simulink library "ECGAnalysisLib"  (R2020b)
settings: Solver=VariableStepAuto  StartTime=0.0  StopTime=10.0  RelTol=1e-3
undefined symbols (not defined in the file or in its folder): fs, max_hr, max_rr_dev
libraries: $bdroot x3
settings Model: Creator=Rafael  LastModifiedBy=Rafael

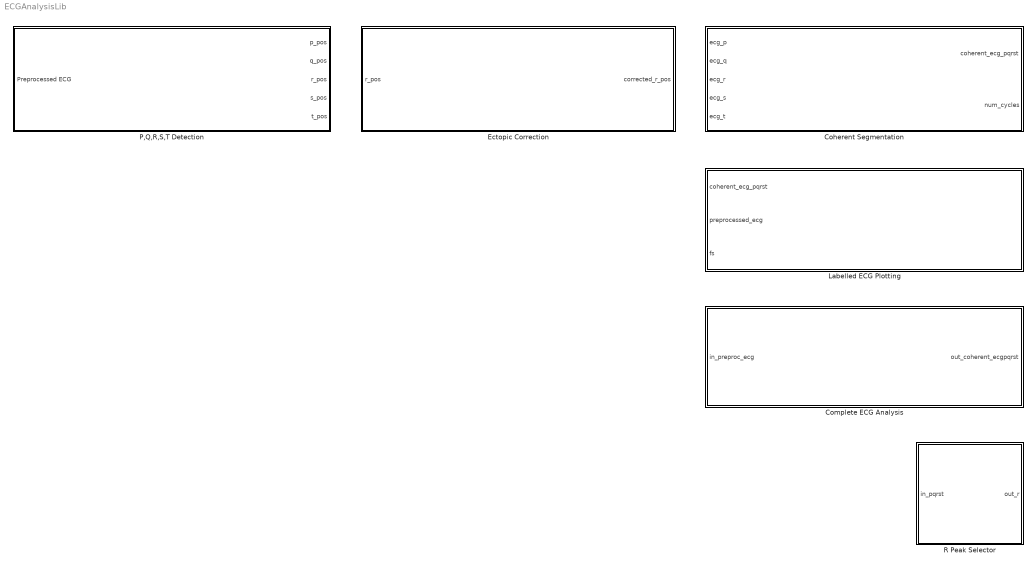
== system ECGAnalysisLib ==
  Coherent Segmentation : Subsystem
      mask Display: image('$imagefile'); % Use "Edit Image" on toolstrip to change.
  Complete ECG Analysis : Subsystem
      mask Display: image('$imagefile'); % Use "Edit Image" on toolstrip to change.
  Ectopic Correction : Subsystem
      mask Display: image('Tachogram.jpg'); % Use "Edit Image" on toolstrip to change.
  Labelled ECG Plotting : MATLAB Function  TreatAsAtomicUnit=on
  P,Q,R,S,T Detection : Subsystem  mask{ecg_algo=PQRST waves - Multi-level Teager Energy Operator}
      mask prompts: ecg_algo "Choose one:"
      mask init:
      | if ecg_algo == 1
      |     param_ecg_algo = 'Pan-Tompkins';
      | elseif ecg_algo == 2
      |     param_ecg_algo = 'Phase Space';
      | elseif ecg_algo == 3
      |     param_ecg_algo = 'Filter Bank';
      | elseif ecg_algo == 4
      |     param_ecg_algo = 'State Machine';
      | elseif ecg_algo == 5
      |     param_ecg_algo = 'Multi-level Teager Energy Operator';
      | end
      | 
      | assignin('base','param_ecg_algo', param_ecg_algo)
      mask TypeOptions ecg_algo: R wave  - Pan-Tompkins | R wave - Phase space | R wave - Filter bank | QRST waves - State machine | PQRST waves - Multi-level Teager Energy Operator
      mask DialogControl DescGroupVar Prompt: ECG PQRST Detection
      mask DialogControl DescTextVar Prompt: Select detected waveform(s) and corresponding detection aglorithm.
      mask DialogControl ParameterGroupVar Prompt: Desired wave(s) and Algorithm
      mask Display: image('$imagefile'); % Use "Edit Image" on toolstrip to change.
  R Peak Selector : Subsystem
      mask Display: image('$imagefile'); % Use "Edit Image" on toolstrip to change.

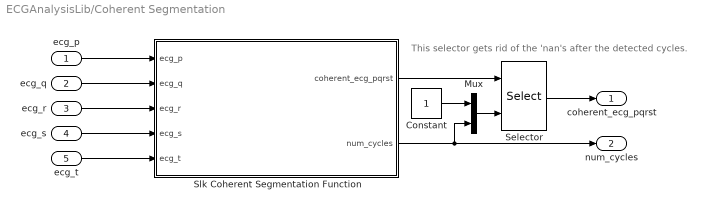
== system ECGAnalysisLib/Coherent Segmentation ==
  note: This selector gets rid of the 'nan's after the detected cycles.
  ecg_p : Inport
  ecg_q : Inport  Port=2
  ecg_r : Inport  Port=3
  ecg_s : Inport  Port=4
  ecg_t : Inport  Port=5
  Constant : Constant
  Mux : Mux  Inputs=2
  Selector : Selector  NumberOfDimensions=2  InputPortWidth=3  IndexOptions=Starting and ending indices (port),Index vector (dialog)  Indices=[1 3],[1 2 3 3 5]  OutputSizes=1,1
  Slk Coherent Segmentation Function : MATLAB Function  TreatAsAtomicUnit=on
  coherent_ecg_pqrst : Outport
  num_cycles : Outport  Port=2
  wires:
  ecg_q/1 -> Slk Coherent Segmentation Function/2(ecg_q)
  ecg_s/1 -> Slk Coherent Segmentation Function/4(ecg_s)
  ecg_p/1 -> Slk Coherent Segmentation Function/1(ecg_p)
  ecg_r/1 -> Slk Coherent Segmentation Function/3(ecg_r)
  ecg_t/1 -> Slk Coherent Segmentation Function/5(ecg_t)
  Constant/1 -> Mux/1
  Mux/1 -> Selector/2
  Slk Coherent Segmentation Function/1(coherent_ecg_pqrst) -> Selector/1
  Selector/1 -> coherent_ecg_pqrst/1
  Slk Coherent Segmentation Function/2(num_cycles) -> num_cycles/1, Mux/2

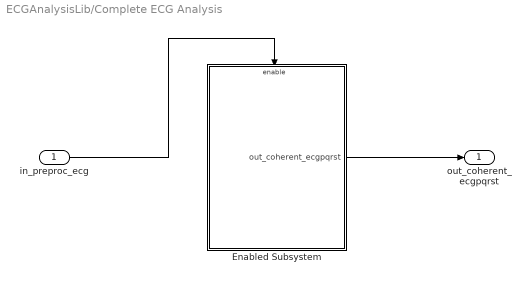
== system ECGAnalysisLib/Complete ECG Analysis ==
  in_preproc_ecg : Inport
  Enabled Subsystem : Subsystem  TreatAsAtomicUnit=on
  out_coherent_ecgpqrst : Outport
  wires:
  Enabled Subsystem/1(out_coherent_ecgpqrst) -> out_coherent_ecgpqrst/1
  in_preproc_ecg/1 -> Enabled Subsystem/Enable

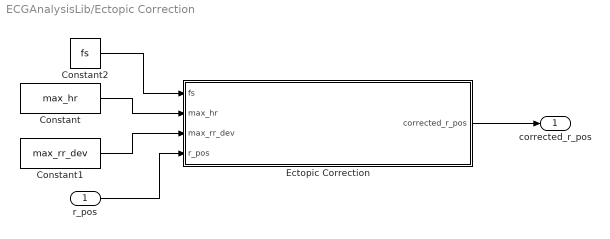
== system ECGAnalysisLib/Ectopic Correction ==
  r_pos : Inport
  Constant : Constant  Value=max_hr
  Constant1 : Constant  Value=max_rr_dev
  Constant2 : Constant  Value=fs
  Ectopic Correction : MATLAB Function  TreatAsAtomicUnit=on
  corrected_r_pos : Outport
  wires:
  r_pos/1 -> Ectopic Correction/4(r_pos)
  Ectopic Correction/1(corrected_r_pos) -> corrected_r_pos/1
  Constant2/1 -> Ectopic Correction/1(fs)
  Constant/1 -> Ectopic Correction/2(max_hr)
  Constant1/1 -> Ectopic Correction/3(max_rr_dev)

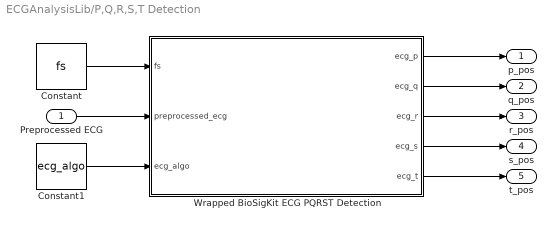
== system ECGAnalysisLib/P,Q,R,S,T Detection ==
  Preprocessed ECG : Inport
  Constant : Constant  Value=fs
  Constant1 : Constant  Value=ecg_algo
  Wrapped BioSigKit ECG PQRST Detection : MATLAB Function  TreatAsAtomicUnit=on
  p_pos : Outport
      settings: VarSizeSig=Yes
  q_pos : Outport  Port=2
      settings: VarSizeSig=Yes
  r_pos : Outport  Port=3
      settings: VarSizeSig=Yes
  s_pos : Outport  Port=4
      settings: VarSizeSig=Yes
  t_pos : Outport  Port=5
      settings: VarSizeSig=Yes
  wires:
  Preprocessed ECG/1 -> Wrapped BioSigKit ECG PQRST Detection/2(preprocessed_ecg)
  Constant/1 -> Wrapped BioSigKit ECG PQRST Detection/1(fs)
  Wrapped BioSigKit ECG PQRST Detection/1(ecg_p) -> p_pos/1
  Wrapped BioSigKit ECG PQRST Detection/2(ecg_q) -> q_pos/1
  Wrapped BioSigKit ECG PQRST Detection/3(ecg_r) -> r_pos/1
  Wrapped BioSigKit ECG PQRST Detection/4(ecg_s) -> s_pos/1
  Wrapped BioSigKit ECG PQRST Detection/5(ecg_t) -> t_pos/1
  Constant1/1 -> Wrapped BioSigKit ECG PQRST Detection/3(ecg_algo)

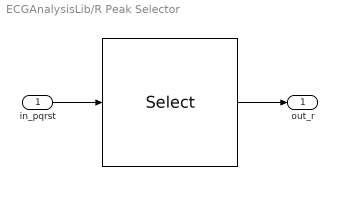
== system ECGAnalysisLib/R Peak Selector ==
  in_pqrst : Inport
  " " : Selector  NumberOfDimensions=2  InputPortWidth=3  IndexOptions=Select all,Index vector (dialog)  Indices=[1 3],3  OutputSizes=1,1
  out_r : Outport
  wires:
  in_pqrst/1 -> " "/1
  " "/1 -> out_r/1

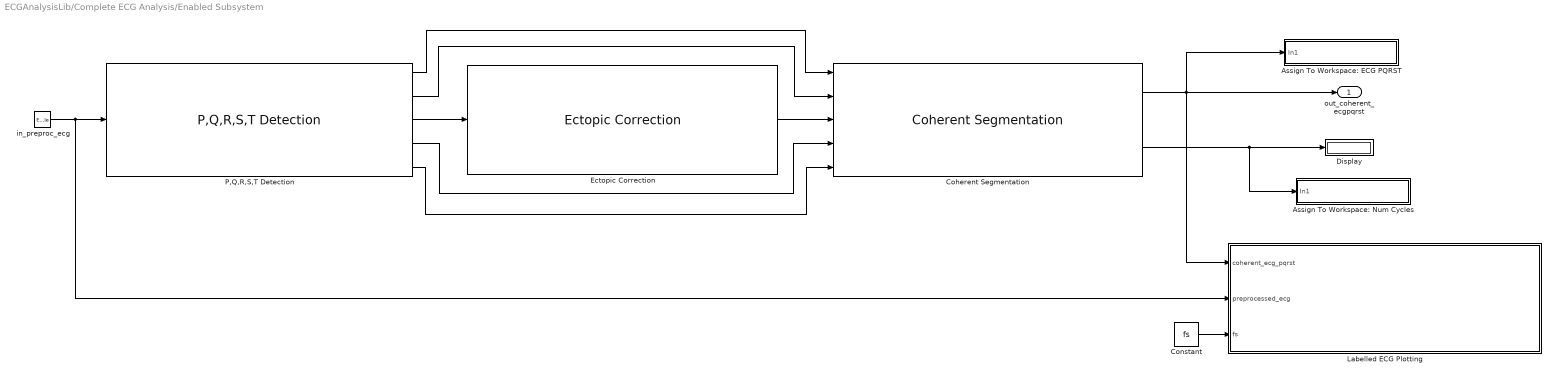
== system ECGAnalysisLib/Complete ECG Analysis/Enabled Subsystem ==
  in_preproc_ecg : EnablePort  ShowOutputPort=on
  Assign To Workspace: ECG PQRST : Subsystem
      mask Display: disp('Assign: out_ecg_pqrst')
  Assign To Workspace: Num Cycles : Subsystem
      mask Display: disp('Assign: out_ecg_num_cycles')
  Coherent Segmentation : $bdroot/Coherent Segmentation  SystemSampleTime=-1  VariantActivationTime=update diagram  Latency=0  AutoFrameSizeCalculation=off
  Constant : Constant  Value=fs
  Display : Display
  Ectopic Correction : $bdroot/Ectopic Correction  SystemSampleTime=-1  VariantActivationTime=update diagram  Latency=0  AutoFrameSizeCalculation=off
  Labelled ECG Plotting : MATLAB Function  TreatAsAtomicUnit=on
  P,Q,R,S,T Detection : $bdroot/P,Q,R,S,T Detection  ecg_algo=PQRST waves - Multi-level Teager Energy Operator
  out_coherent_ecgpqrst : Outport
  wires:
  P,Q,R,S,T Detection/3 -> Ectopic Correction/1
  Ectopic Correction/1 -> Coherent Segmentation/3
  P,Q,R,S,T Detection/1 -> Coherent Segmentation/1
  P,Q,R,S,T Detection/2 -> Coherent Segmentation/2
  P,Q,R,S,T Detection/4 -> Coherent Segmentation/4
  P,Q,R,S,T Detection/5 -> Coherent Segmentation/5
  in_preproc_ecg/1 -> Labelled ECG Plotting/2(preprocessed_ecg), P,Q,R,S,T Detection/1
  Constant/1 -> Labelled ECG Plotting/3(fs)
  Coherent Segmentation/1 -> Assign To Workspace: ECG PQRST/1(In1), Labelled ECG Plotting/1(coherent_ecg_pqrst), out_coherent_ecgpqrst/1
  Coherent Segmentation/2 -> Assign To Workspace: Num Cycles/1(In1), Display/1

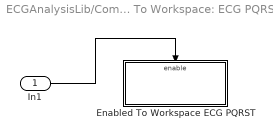
== system ECGAnalysisLib/Complete ECG Analysis/Enabled Subsystem/Assign To Workspace: ECG PQRST ==
  In1 : Inport
  Enabled To Workspace ECG PQRST : Subsystem  TreatAsAtomicUnit=on
  wires:
  In1/1 -> Enabled To Workspace ECG PQRST/Enable

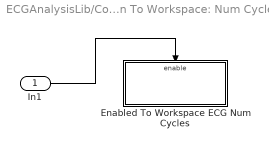
== system ECGAnalysisLib/Complete ECG Analysis/Enabled Subsystem/Assign To Workspace: Num Cycles ==
  In1 : Inport
  Enabled To Workspace ECG Num Cycles : Subsystem  TreatAsAtomicUnit=on
  wires:
  In1/1 -> Enabled To Workspace ECG Num Cycles/Enable

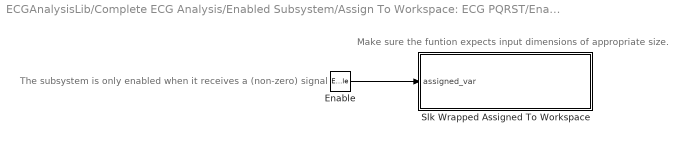
== system ECGAnalysisLib/Complete ECG Analysis/Enabled Subsystem/Assign To Workspace: ECG PQRST/Enabled To Workspace ECG PQRST ==
  note: Make sure the funtion expects input dimensions of appropriate size.
  note: The subsystem is only enabled when it receives a (non-zero) signal
  Enable : EnablePort  ShowOutputPort=on
  Slk Wrapped Assigned To Workspace : MATLAB Function  TreatAsAtomicUnit=on
  wires:
  Enable/1 -> Slk Wrapped Assigned To Workspace/1(assigned_var)

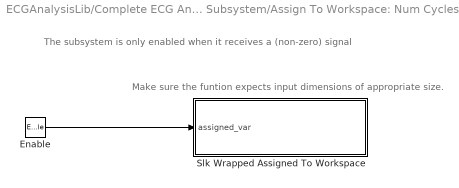
== system ECGAnalysisLib/Complete ECG Analysis/Enabled Subsystem/Assign To Workspace: Num Cycles/Enabled To Workspace ECG Num Cycles ==
  note: The subsystem is only enabled when it receives a (non-zero) signal
  note: Make sure the funtion expects input dimensions of appropriate size.
  Enable : EnablePort  ShowOutputPort=on
  Slk Wrapped Assigned To Workspace : MATLAB Function  TreatAsAtomicUnit=on
  wires:
  Enable/1 -> Slk Wrapped Assigned To Workspace/1(assigned_var)

== matlab function ECGAnalysisLib/Coherent Segmentation/Slk Coherent Segmentation Function ==
  data: ecg_p input size=[4*ceil(param_sim_time) 1]; coherent_ecg_pqrst output size=[4*ceil(param_sim_time) 5]; ecg_q input size=[4*ceil(param_sim_time) 1]; ecg_r input size=[4*ceil(param_sim_time) 1]; ecg_s input size=[4*ceil(param_sim_time) 1]; ecg_t input size=[4*ceil(param_sim_time) 1]; num_cycles output size=1
function [coherent_ecg_pqrst, num_cycles] = slk_coherent_segmentation(ecg_p, ecg_q, ecg_r, ecg_s, ecg_t)
% Function to associate the detected PQRST peaks to each other in a
% coherent way. The function will produce an output 'coherent_ecg_pqrst' of
% size [num_cycles x 5]. The 5 corresponds to the 5 fiducial points (PQRST
% peaks). num_cycles is the number of detected R peaks (heart cycles). The
% first column of coherent_ecg_prqst corresponds to the detected P waves,
% where the row corresponds to that cycle number. If a P wave couldnt be
% detected for that cycle, it is replaced with 'Nan'.


if ecg_r % Only go into the function if a valid ecg R peak sequence is passed to it.
    
    % Preinitialization.
    coherent_ecg_p = zeros(length(ecg_r),1);
    coherent_ecg_q = zeros(length(ecg_r),1);
    coherent_ecg_r = zeros(length(ecg_r),1);
    coherent_ecg_s = zeros(length(ecg_r),1);
    coherent_ecg_t = zeros(length(ecg_r),1);
        
    %% First Cycle.
    
    % P Wave.
    temp = ecg_p(find(ecg_p < ecg_r(1)));
    if isempty(temp)
        coherent_ecg_p(1) = nan;
        temp = [];
    else
        coherent_ecg_p(1) = temp;
    end
    
    % Q Wave.
    temp = ecg_p(find(ecg_q < ecg_r(1)));
    if isempty(temp)
        coherent_ecg_q(1) = nan;
        temp = [];
    else
        coherent_ecg_q(1) = temp;
    end
    
    % R Wave.
    coherent_ecg_r(1) = ecg_r(1);
    
    % S Wave.
    temp = ecg_s(find(ecg_s > ecg_r(1) & ecg_s < ecg_r(2)));
    if isempty(temp)
        coherent_ecg_s(1) = nan;
        temp = [];
    else
        coherent_ecg_s(1) = temp;
    end
    
    % T Wave.
    temp = ecg_t(find(ecg_t > ecg_r(1) & ecg_t < ecg_r(2)));
    if isempty(temp)
        coherent_ecg_t(1) = nan;
        temp = [];
    else
        coherent_ecg_t(1) = temp;
    end
    
    %% Cycle 2:End-1.
    for i = 2:length(ecg_r)-1
        
        % P Wave.
        temp = ecg_p(find(ecg_p > ecg_r(i-1) & ecg_p < ecg_r(i)));
        if isempty(temp) || length(temp) > 1
            coherent_ecg_p(i) = nan;
            temp = [];
        else
            coherent_ecg_p(i) = temp;
        end
        
        % Q Wave.
        temp = ecg_q(find(ecg_q > ecg_r(i-1) & ecg_q < ecg_r(i)));
        if isempty(temp) || length(temp) > 1
            coherent_ecg_q(i) = nan;
            temp = [];
        else
            coherent_ecg_q(i) = temp;
        end
        
        % R Wave.
        coherent_ecg_r(i) = ecg_r(i);
        
        % S Wave.
        temp = ecg_s(find(ecg_s > ecg_r(i) & ecg_s < ecg_r(i+1)));
        if isempty(temp) || length(temp) > 1
            coherent_ecg_s(i) = nan;
            temp = [];
        else
            coherent_ecg_s(i) = temp;
        end
        
        % T Wave.
        temp = ecg_t(find(ecg_t > ecg_r(i) & ecg_t < ecg_r(i+1)));
        if isempty(temp) || length(temp) > 1
            coherent_ecg_t(i) = nan;
            temp = [];
        else
            coherent_ecg_t(i) = temp;
        end
    end
    
    %% Last Cycle.
    
    % P Wave.
    temp = ecg_p(find(ecg_p > ecg_r(end-1) & ecg_p < ecg_r(end)));
    if isempty(temp) || length(temp) > 1
        coherent_ecg_p(length(ecg_r)) = nan;
        temp = [];
    else
        coherent_ecg_p(length(ecg_r)) = temp;
    end
    
    % Q Wave.
    temp = ecg_q(find(ecg_q > ecg_r(end-1) & ecg_q < ecg_r(end)));
    if isempty(temp) || length(temp) > 1
        coherent_ecg_q(length(ecg_r)) = nan;
        temp = [];
    else
        coherent_ecg_q(length(ecg_r)) = temp;
    end
    
    % R Wave.
    coherent_ecg_r(length(ecg_r)) = ecg_r(length(ecg_r));
    
    % S Wave.
    temp = ecg_s(find(ecg_s > ecg_r(1) & ecg_s < ecg_r(2)));
    if isempty(temp) || length(temp) > 1
        coherent_ecg_s(length(ecg_r)) = nan;
        temp = [];
    else
        coherent_ecg_s(length(ecg_r)) = temp;
    end
    
    % T Wave.
    temp = ecg_t(find(ecg_t > ecg_r(1) & ecg_t < ecg_r(2)));
    if isempty(temp) || length(temp) > 1
        coherent_ecg_t(length(ecg_r)) = nan;
        temp = [];
    else
        coherent_ecg_t(length(ecg_r)) = temp;
    end
    
    coherent_ecg_pqrst = [coherent_ecg_p coherent_ecg_q coherent_ecg_r coherent_ecg_s coherent_ecg_t];
    num_cycles = length(coherent_ecg_r);  
    
else
    
    coherent_ecg_pqrst = [];
    num_cycles = 0;
end
end

== matlab function ECGAnalysisLib/Labelled ECG Plotting ==
  data: coherent_ecg_pqrst input size=[4*ceil(param_sim_time) 5]; preprocessed_ecg input size=[param_tot_samples 1]; fs input size=[1]
function slk_wrapped_plotting_ecg_pqrst(coherent_ecg_pqrst, preprocessed_ecg, fs)
    
coder.extrinsic('plotting_ecg_pqrst');

if coherent_ecg_pqrst(:,3) % Only go into the function if a valid ecg R peak sequence is passed to it.
    plotting_ecg_pqrst(coherent_ecg_pqrst, preprocessed_ecg, fs)
end

end

== matlab function ECGAnalysisLib/Complete ECG Analysis/Enabled Subsystem/Labelled ECG Plotting ==
  data: coherent_ecg_pqrst input size=[4*ceil(param_sim_time) 5]; preprocessed_ecg input size=[param_tot_samples 1]; fs input size=[1]
function slk_wrapped_plotting_ecg_pqrst(coherent_ecg_pqrst, preprocessed_ecg, fs)
    
coder.extrinsic('plotting_ecg_pqrst');

if coherent_ecg_pqrst(:,3) % Only go into the function if a valid ecg R peak sequence is passed to it.
    plotting_ecg_pqrst(coherent_ecg_pqrst, preprocessed_ecg, fs)
end

end

== matlab function ECGAnalysisLib/Complete ECG Analysis/Enabled Subsystem/Assign To Workspace: ECG PQRST/Enabled To Workspace ECG PQRST/Slk Wrapped Assigned To Workspace ==
  data: assigned_var input size=[1]
function slk_wrapped_assign_to_workspace(assigned_var)
% Wrapped simulink function to assign an input 'assigned_var' to the base workspace.

coder.extrinsic('assign_num_cycles_to_workspace');

if assigned_var % Only go into the function if a valid variable is passed to it.
    assign_num_cycles_to_workspace(assigned_var)
end

end

== matlab function ECGAnalysisLib/P,Q,R,S,T Detection/Wrapped BioSigKit ECG PQRST Detection ==
  data: ecg_p output size=[4*ceil(param_sim_time) 1]; ecg_q output size=[4*ceil(param_sim_time) 1]; ecg_r output size=[4*ceil(param_sim_time) 1]; ecg_s output size=[4*ceil(param_sim_time) 1]; ecg_t output size=[4*ceil(param_sim_time) 1]; fs input; preprocessed_ecg input; ecg_algo input
function [ecg_p, ecg_q, ecg_r, ecg_s, ecg_t] = slk_wrapped_BioSigKit_ECG_Detection(fs, preprocessed_ecg, ecg_algo)

% This function is split in two parts out of necessity - (Simulink is kind of dumb).
% The first part counts how many detected P,Q,R,S, and T waves there are according to the BioSigKit method.
% With these numbers we can pre-initialize the size of the vectors holding the sample positions of these P,Q,R,S, and T waves which are then
% identified using a second identical use of the BioSigKit detection method.

coder.extrinsic('BioSigKit_ECG_Count_Detection');
coder.extrinsic('BioSigKit_ECG_Peak_Detection');

if preprocessed_ecg % The function is only run if a non-zero signal is passed to it.
    %% Part 1 - P,Q,R,S,T Count
    num_p = -1; % Pre-Initialization.
    num_q = -1;
    num_r = -1;
    num_s = -1;
    num_t = -1;
    
    [num_p, num_q, num_r, num_s, num_t] = BioSigKit_ECG_Count_Detection(fs,preprocessed_ecg, ecg_algo);
    
    %% Part 2 - P,Q,R,S,T Peak Identification
    ecg_p = zeros(num_p,1); % Pre-Initialization.
    ecg_q = zeros(num_q,1);
    ecg_r = zeros(num_r,1);
    ecg_s = zeros(num_s,1);
    ecg_t = zeros(num_t,1);
    
    % Performing the detection according to the desired detection algorithm.
    if ecg_algo == 1  || ecg_algo == 2 || ecg_algo == 3
        
        [~, ~, ecg_r(1:num_r), ~, ~] = BioSigKit_ECG_Peak_Detection(fs,preprocessed_ecg, ecg_algo);
        ecg_p = nan; ecg_q = nan; ecg_s = nan; ecg_t = nan;
        
    elseif ecg_algo == 4
        
        [~, ecg_q(1:num_q), ecg_r(1:num_r), ecg_s(1:num_s), ecg_t(1:num_t)] = BioSigKit_ECG_Peak_Detection(fs,preprocessed_ecg, ecg_algo);
        ecg_p = nan;
        
    elseif ecg_algo == 5
        
        [ecg_p(1:num_p), ecg_q(1:num_q), ecg_r(1:num_r), ecg_s(1:num_s), ecg_t(1:num_t)] = BioSigKit_ECG_Peak_Detection(fs,preprocessed_ecg, ecg_algo);
        
    end
        
else % If there's no input - pass an empty output.
    
    ecg_p = [];
    ecg_q = [];
    ecg_r = [];
    ecg_s = [];
    ecg_t = [];
    
end

== matlab function ECGAnalysisLib/Ectopic Correction/Ectopic Correction ==
  data: fs input; max_hr input; max_rr_dev input; r_pos input size=[4*ceil(param_sim_time) 1]; corrected_r_pos output size=[4*ceil(param_sim_time) 1]
function corrected_r_pos = slk_ectopic_correction(fs, max_hr, max_rr_dev, r_pos)

if r_pos % Only run if a series of R peaks are passed.
    
    corrected_r_pos = r_pos;
    
    rr = diff(r_pos); % RR interval calculation.
    
    %% Part 1 - Identification of Cycles over the Maximum Heart Rate.
    max_rr_sec = 1/(max_hr/60); % In sec.
    max_rr_samples = max_rr_sec*fs; % In samples.
    
    tachogram = 60./(rr/fs); % Tachogram calculation (in bpm).
    
    % Plotting the tachogram.
    fig_tachogram = figure;
    plot(r_pos(1:end-1)/fs,tachogram); title('Tachogram'); xlabel('R Time (sec)'); ylabel('Heart Rate (bpm)'); box off; hold on;
    line([0 r_pos(end-1)/fs],[max_hr max_hr],'Color','red','LineStyle','--'); hold on
    
    % Identifying the ectopies faster than the Maximum Heart Rate threshold and labelling them as 'nan'.
    ectopies_1 = find(rr < max_rr_samples);
    rr(ectopies_1) = nan;
    r_pos(ectopies_1 + 1) = nan;
    
    %% Part 2 - Identification of Cycles over the RR Deviation Threshold.    
    % Evaluating the adaptive RR deviation threshold (a 7-cycle moving median). The detected ectopies of part 1 do not compute for this moving median.
    plot_thr = 60./(movmedian(rr,7,'omitnan')/fs) + max_rr_dev; % The threshold to be plotted on the tachogram (in bpm).
    thr = fs./(plot_thr/60); % The equivalent threshold in samples - to be compared against the calculated RR intervals.
    
    % Plotting the adaptive threshold on the tachogram.
    plot(r_pos(1:end-1)/fs,plot_thr,'r--'); hold on;
    
    % Identifying Ectopies
    ectopies_2 = find(thr - rr > 0 );
    
    %% Part 3 - Labelling and removing the detected ectopies.

    ectopies = [ectopies_1; ectopies_2];
    ectopies = sort(ectopies);
    
    plot(r_pos(ectopies)/fs,tachogram(ectopies),'ro'); hold on; 
    corrected_r_pos(ectopies) = [];
   
else
    corrected_r_pos = r_pos;
end

end

== matlab function ECGAnalysisLib/Complete ECG Analysis/Enabled Subsystem/Assign To Workspace: Num Cycles/Enabled To Workspace ECG Num Cycles/Slk Wrapped Assigned To Workspace ==
  data: assigned_var input size=[1]
function slk_wrapped_assign_to_workspace(assigned_var)
% Wrapped simulink function to assign an input 'assigned_var' to the base workspace.

coder.extrinsic('assign_num_cycles_to_workspace');

if assigned_var % Only go into the function if a valid variable is passed to it.
    assign_num_cycles_to_workspace(assigned_var)
end

end
